simulink model "ejh68a"  (Simulink 3.00)
settings: Solver=ode5  StartTime=0.0  StopTime=30.0  FixedStep=0.1  MaxStep=0.001  RelTol=1e-3
undefined symbols (not defined in the file or in its folder): nonlinear
settings Model: LastModifiedBy=Administrador

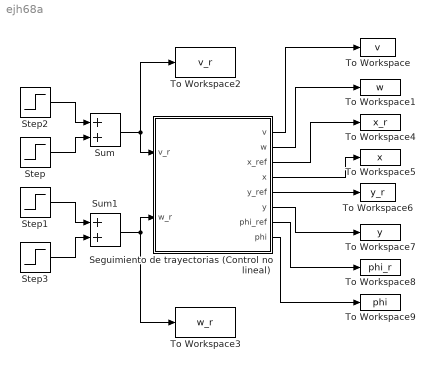
== system ejh68a ==
  Seguimiento de trayectorias (Control no lineal) : Subsystem  mask(Seguimiento de trayectorias empleando una ley de control no lineal){b=13.75, d=0.9, K2=19, x_inicial=1, y_inicial=0.5, phi_inicial=pi/6, x_r_inicial=0, y_r_inicial=0, phi_r_inicial=0}
      mask prompts: b "Parámetro beta:"; d "Parámetro delta:"; K2 "Parámetro K2:"; x_inicial "Coordenada x inicial del robot:"; y_inicial "Coordenada y inicial del robot:"; phi_inicial "Valor inicial de la orientación del robot (rad):"; x_r_inicial "Coordenada x inicial de la referencia:"; y_r_inicial "Coordenada y inicial de la referencia:"; phi_r_inicial "Orientación inicial de la referencia (rad):"
      mask help:
      | Este bloque permite simular una estrategia de control no lineal para el seguimiento de trayectorias. A la entrada se dispone de las velocidades lineal y angular de referencia. Se supone un cierto modelo para el vehículo.
      | El usuario puede modificar este bloque para introducir como referencia las coordenadas (x,y) y la orientación deseadas.
  Step : Step  Time=0  Before=0  After=0.2  SampleTime=0
  Step1 : Step  Time=0  Before=0  After=0.3  SampleTime=0
  Step2 : Step  Time=20  Before=0  After=-0.1  SampleTime=0
  Step3 : Step  Time=10  Before=0  After=-0.1  SampleTime=0
  Sum : Sum  Inputs=++  SaturateOnIntegerOverflow=on
  Sum1 : Sum  Inputs=++  SaturateOnIntegerOverflow=on
  To Workspace : ToWorkspace  VariableName=v  SampleTime=-1  SaveFormat=Matrix
  To Workspace1 : ToWorkspace  VariableName=w  SampleTime=-1  SaveFormat=Matrix
  To Workspace2 : ToWorkspace  VariableName=v_r  SampleTime=-1  SaveFormat=Matrix
  To Workspace3 : ToWorkspace  VariableName=w_r  SampleTime=-1  SaveFormat=Matrix
  To Workspace4 : ToWorkspace  VariableName=x_r  SampleTime=-1  SaveFormat=Matrix
  To Workspace5 : ToWorkspace  VariableName=x  SampleTime=-1  SaveFormat=Matrix
  To Workspace6 : ToWorkspace  VariableName=y_r  SampleTime=-1  SaveFormat=Matrix
  To Workspace7 : ToWorkspace  VariableName=y  SampleTime=-1  SaveFormat=Matrix
  To Workspace8 : ToWorkspace  VariableName=phi_r  SampleTime=-1  SaveFormat=Matrix
  To Workspace9 : ToWorkspace  VariableName=phi  SampleTime=-1  SaveFormat=Matrix
  wires:
  Step2/1 -> Sum/1
  Step/1 -> Sum/2
  Step1/1 -> Sum1/1
  Step3/1 -> Sum1/2
  Sum1/1 -> To Workspace3/1, Seguimiento de trayectorias (Control no lineal)/2(w_r)
  Sum/1 -> To Workspace2/1, Seguimiento de trayectorias (Control no lineal)/1(v_r)
  Seguimiento de trayectorias (Control no lineal)/1(v) -> To Workspace/1
  Seguimiento de trayectorias (Control no lineal)/2(w) -> To Workspace1/1
  Seguimiento de trayectorias (Control no lineal)/3(x_ref) -> To Workspace4/1
  Seguimiento de trayectorias (Control no lineal)/5(y_ref) -> To Workspace6/1
  Seguimiento de trayectorias (Control no lineal)/6(y) -> To Workspace7/1
  Seguimiento de trayectorias (Control no lineal)/7(phi_ref) -> To Workspace8/1
  Seguimiento de trayectorias (Control no lineal)/4(x) -> To Workspace5/1
  Seguimiento de trayectorias (Control no lineal)/8(phi) -> To Workspace9/1

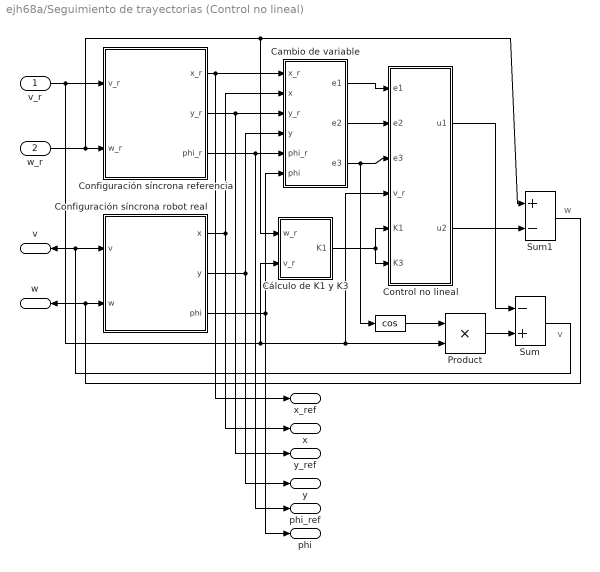
== system ejh68a/Seguimiento de trayectorias (Control no lineal) ==
  note: v
  note: w
  v_r : Inport  Port=1  PortWidth=-1  SampleTime=-1  DataType=auto
      settings: SignalType=auto
  w_r : Inport  Port=2  PortWidth=-1  SampleTime=-1  DataType=auto
      settings: SignalType=auto
  " " : Trigonometry  Operator=cos  OutputSignalType=auto
  Cambio de variable : Subsystem
  Configuración síncrona referencia : Subsystem
  Configuración síncrona robot real : Subsystem
  Control no lineal : Subsystem
  Cálculo de K1 y K3 : Subsystem
  Product : Product  Inputs=2  SaturateOnIntegerOverflow=on
  Sum : Sum  Inputs=-+  SaturateOnIntegerOverflow=on
  Sum1 : Sum  Inputs=+-  SaturateOnIntegerOverflow=on
  v : Outport  Orientation=left  Port=1
  w : Outport  Orientation=left  Port=2
  x_ref : Outport  Port=3
  x : Outport  Port=4
  y_ref : Outport  Port=5
  y : Outport  Port=6
  phi_ref : Outport  Port=7
  phi : Outport  Port=8
  wires:
  v_r/1 -> Configuración síncrona referencia/1(v_r), Product/2, Control no lineal/4(v_r), Cálculo de K1 y K3/2(v_r)
  " "/1 -> Product/1
  Product/1 -> Sum/2
  w_r/1 -> Configuración síncrona referencia/2(w_r), Sum1/1, Cálculo de K1 y K3/1(w_r)
  Sum1/1 -> Configuración síncrona robot real/2(w), w/1
  Sum/1 -> Configuración síncrona robot real/1(v), v/1
  Control no lineal/2(u2) -> Sum1/2
  Control no lineal/1(u1) -> Sum/1
  Cambio de variable/1(e1) -> Control no lineal/1(e1)
  Cambio de variable/2(e2) -> Control no lineal/2(e2)
  Cambio de variable/3(e3) -> " "/1, Control no lineal/3(e3)
  Cálculo de K1 y K3/1(K1) -> Control no lineal/5(K1), Control no lineal/6(K3)
  Configuración síncrona robot real/3(phi) -> Cambio de variable/6(phi), phi/1
  Configuración síncrona referencia/1(x_r) -> Cambio de variable/1(x_r), x_ref/1
  Configuración síncrona robot real/1(x) -> Cambio de variable/2(x), x/1
  Configuración síncrona referencia/2(y_r) -> Cambio de variable/3(y_r), y_ref/1
  Configuración síncrona robot real/2(y) -> Cambio de variable/4(y), y/1
  Configuración síncrona referencia/3(phi_r) -> Cambio de variable/5(phi_r), phi_ref/1

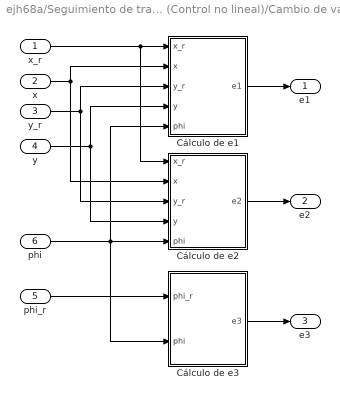
== system ejh68a/Seguimiento de trayectorias (Control no lineal)/Cambio de variable ==
  x_r : Inport  Port=1  PortWidth=-1  SampleTime=-1  DataType=auto
      settings: SignalType=auto
  x : Inport  Port=2  PortWidth=-1  SampleTime=-1  DataType=auto
      settings: SignalType=auto
  y_r : Inport  Port=3  PortWidth=-1  SampleTime=-1  DataType=auto
      settings: SignalType=auto
  y : Inport  Port=4  PortWidth=-1  SampleTime=-1  DataType=auto
      settings: SignalType=auto
  phi_r : Inport  Port=5  PortWidth=-1  SampleTime=-1  DataType=auto
      settings: SignalType=auto
  phi : Inport  Port=6  PortWidth=-1  SampleTime=-1  DataType=auto
      settings: SignalType=auto
  Cálculo de e1 : Subsystem
  Cálculo de e2 : Subsystem
  Cálculo de e3 : Subsystem
  e1 : Outport  Port=1
  e2 : Outport  Port=2
  e3 : Outport  Port=3
  wires:
  x_r/1 -> Cálculo de e1/1(x_r), Cálculo de e2/1(x_r)
  x/1 -> Cálculo de e1/2(x), Cálculo de e2/2(x)
  y_r/1 -> Cálculo de e1/3(y_r), Cálculo de e2/3(y_r)
  y/1 -> Cálculo de e1/4(y), Cálculo de e2/4(y)
  phi_r/1 -> Cálculo de e3/1(phi_r)
  phi/1 -> Cálculo de e2/5(phi), Cálculo de e3/2(phi), Cálculo de e1/5(phi)
  Cálculo de e1/1(e1) -> e1/1
  Cálculo de e2/1(e2) -> e2/1
  Cálculo de e3/1(e3) -> e3/1

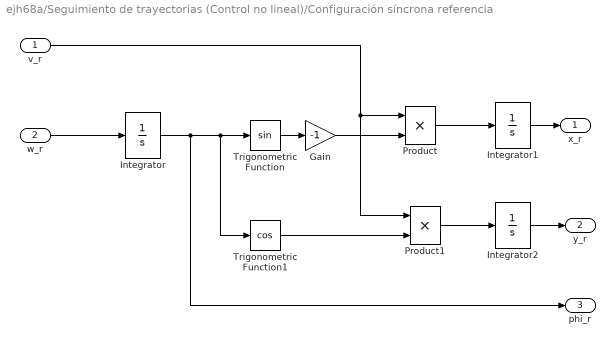
== system ejh68a/Seguimiento de trayectorias (Control no lineal)/Configuración síncrona referencia ==
  v_r : Inport  Port=1  PortWidth=-1  SampleTime=-1  DataType=auto
      settings: SignalType=auto
  w_r : Inport  Port=2  PortWidth=-1  SampleTime=-1  DataType=auto
      settings: SignalType=auto
  Gain : Gain  Gain=-1  SaturateOnIntegerOverflow=on
  Integrator : Integrator  ExternalReset=none  InitialConditionSource=internal  InitialCondition=phi_r_inicial  LimitOutput=off  UpperSaturationLimit=inf  LowerSaturationLimit=-inf  ShowSaturationPort=off  ShowStatePort=off  AbsoluteTolerance=auto
  Integrator1 : Integrator  ExternalReset=none  InitialConditionSource=internal  InitialCondition=x_r_inicial  LimitOutput=off  UpperSaturationLimit=inf  LowerSaturationLimit=-inf  ShowSaturationPort=off  ShowStatePort=off  AbsoluteTolerance=auto
  Integrator2 : Integrator  ExternalReset=none  InitialConditionSource=internal  InitialCondition=y_r_inicial  LimitOutput=off  UpperSaturationLimit=inf  LowerSaturationLimit=-inf  ShowSaturationPort=off  ShowStatePort=off  AbsoluteTolerance=auto
  Product : Product  Inputs=2  SaturateOnIntegerOverflow=on
  Product1 : Product  Inputs=2  SaturateOnIntegerOverflow=on
  Trigonometric Function : Trigonometry  Operator=sin  OutputSignalType=auto
  Trigonometric Function1 : Trigonometry  Operator=cos  OutputSignalType=auto
  x_r : Outport  Port=1
  y_r : Outport  Port=2
  phi_r : Outport  Port=3
  wires:
  Product1/1 -> Integrator2/1
  Product/1 -> Integrator1/1
  Integrator/1 -> Trigonometric Function/1, Trigonometric Function1/1, phi_r/1
  Integrator1/1 -> x_r/1
  Integrator2/1 -> y_r/1
  v_r/1 -> Product/1, Product1/1
  w_r/1 -> Integrator/1
  Gain/1 -> Product/2
  Trigonometric Function/1 -> Gain/1
  Trigonometric Function1/1 -> Product1/2

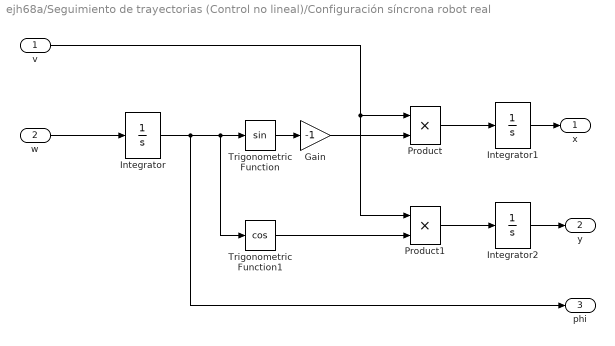
== system ejh68a/Seguimiento de trayectorias (Control no lineal)/Configuración síncrona robot real ==
  v : Inport  Port=1  PortWidth=-1  SampleTime=-1  DataType=auto
      settings: SignalType=auto
  w : Inport  Port=2  PortWidth=-1  SampleTime=-1  DataType=auto
      settings: SignalType=auto
  Gain : Gain  Gain=-1  SaturateOnIntegerOverflow=on
  Integrator : Integrator  ExternalReset=none  InitialConditionSource=internal  InitialCondition=phi_inicial  LimitOutput=off  UpperSaturationLimit=inf  LowerSaturationLimit=-inf  ShowSaturationPort=off  ShowStatePort=off  AbsoluteTolerance=auto
  Integrator1 : Integrator  ExternalReset=none  InitialConditionSource=internal  InitialCondition=x_inicial  LimitOutput=off  UpperSaturationLimit=inf  LowerSaturationLimit=-inf  ShowSaturationPort=off  ShowStatePort=off  AbsoluteTolerance=auto
  Integrator2 : Integrator  ExternalReset=none  InitialConditionSource=internal  InitialCondition=y_inicial  LimitOutput=off  UpperSaturationLimit=inf  LowerSaturationLimit=-inf  ShowSaturationPort=off  ShowStatePort=off  AbsoluteTolerance=auto
  Product : Product  Inputs=2  SaturateOnIntegerOverflow=on
  Product1 : Product  Inputs=2  SaturateOnIntegerOverflow=on
  Trigonometric Function : Trigonometry  Operator=sin  OutputSignalType=auto
  Trigonometric Function1 : Trigonometry  Operator=cos  OutputSignalType=auto
  x : Outport  Port=1
  y : Outport  Port=2
  phi : Outport  Port=3
  wires:
  Product1/1 -> Integrator2/1
  Product/1 -> Integrator1/1
  Gain/1 -> Product/2
  Integrator/1 -> Trigonometric Function/1, Trigonometric Function1/1, phi/1
  Integrator1/1 -> x/1
  Integrator2/1 -> y/1
  v/1 -> Product/1, Product1/1
  w/1 -> Integrator/1
  Trigonometric Function/1 -> Gain/1
  Trigonometric Function1/1 -> Product1/2

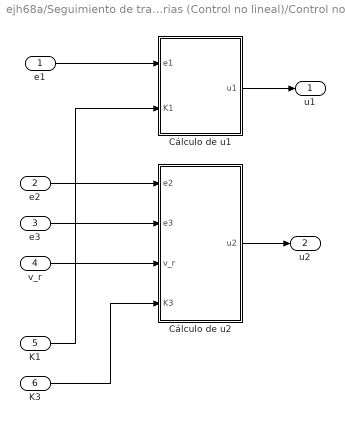
== system ejh68a/Seguimiento de trayectorias (Control no lineal)/Control no lineal ==
  e1 : Inport  Port=1  PortWidth=-1  SampleTime=-1  DataType=auto
      settings: SignalType=auto
  e2 : Inport  Port=2  PortWidth=-1  SampleTime=-1  DataType=auto
      settings: SignalType=auto
  e3 : Inport  Port=3  PortWidth=-1  SampleTime=-1  DataType=auto
      settings: SignalType=auto
  v_r : Inport  Port=4  PortWidth=-1  SampleTime=-1  DataType=auto
      settings: SignalType=auto
  K1 : Inport  Port=5  PortWidth=-1  SampleTime=-1  DataType=auto
      settings: SignalType=auto
  K3 : Inport  Port=6  PortWidth=-1  SampleTime=-1  DataType=auto
      settings: SignalType=auto
  Cálculo de u1 : Subsystem
  "Cálculo de u2 " : Subsystem
  u1 : Outport  Port=1
  u2 : Outport  Port=2
  wires:
  e1/1 -> Cálculo de u1/1(e1)
  e2/1 -> "Cálculo de u2 "/1(e2)
  e3/1 -> "Cálculo de u2 "/2(e3)
  Cálculo de u1/1(u1) -> u1/1
  "Cálculo de u2 "/1(u2) -> u2/1
  v_r/1 -> "Cálculo de u2 "/3(v_r)
  K1/1 -> Cálculo de u1/2(K1)
  K3/1 -> "Cálculo de u2 "/4(K3)

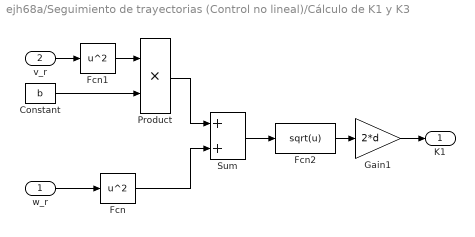
== system ejh68a/Seguimiento de trayectorias (Control no lineal)/Cálculo de K1 y K3 ==
  w_r : Inport  Port=1  PortWidth=-1  SampleTime=-1  DataType=auto
      settings: SignalType=auto
  v_r : Inport  Port=2  PortWidth=-1  SampleTime=-1  DataType=auto
      settings: SignalType=auto
  Constant : Constant  Value=b
  Fcn : Fcn  Expr=u^2
  Fcn1 : Fcn  Expr=u^2
  Fcn2 : Fcn  Expr=sqrt(u)
  Gain1 : Gain  Gain=2*d  SaturateOnIntegerOverflow=on
  Product : Product  Inputs=2  SaturateOnIntegerOverflow=on
  Sum : Sum  Inputs=++  SaturateOnIntegerOverflow=on
  K1 : Outport  Port=1
  wires:
  w_r/1 -> Fcn/1
  v_r/1 -> Fcn1/1
  Fcn1/1 -> Product/1
  Constant/1 -> Product/2
  Product/1 -> Sum/1
  Fcn/1 -> Sum/2
  Sum/1 -> Fcn2/1
  Fcn2/1 -> Gain1/1
  Gain1/1 -> K1/1

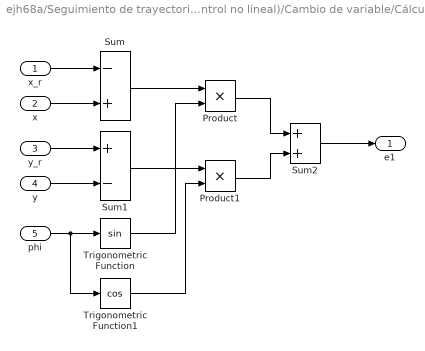
== system ejh68a/Seguimiento de trayectorias (Control no lineal)/Cambio de variable/Cálculo de e1 ==
  x_r : Inport  Port=1  PortWidth=-1  SampleTime=-1  DataType=auto
      settings: SignalType=auto
  x : Inport  Port=2  PortWidth=-1  SampleTime=-1  DataType=auto
      settings: SignalType=auto
  y_r : Inport  Port=3  PortWidth=-1  SampleTime=-1  DataType=auto
      settings: SignalType=auto
  y : Inport  Port=4  PortWidth=-1  SampleTime=-1  DataType=auto
      settings: SignalType=auto
  phi : Inport  Port=5  PortWidth=-1  SampleTime=-1  DataType=auto
      settings: SignalType=auto
  Product : Product  Inputs=2  SaturateOnIntegerOverflow=on
  Product1 : Product  Inputs=2  SaturateOnIntegerOverflow=on
  Sum : Sum  Inputs=-+  SaturateOnIntegerOverflow=on
  Sum1 : Sum  Inputs=+-  SaturateOnIntegerOverflow=on
  Sum2 : Sum  Inputs=++  SaturateOnIntegerOverflow=on
  Trigonometric Function : Trigonometry  Operator=sin  OutputSignalType=auto
  Trigonometric Function1 : Trigonometry  Operator=cos  OutputSignalType=auto
  e1 : Outport  Port=1
  wires:
  x_r/1 -> Sum/1
  x/1 -> Sum/2
  y_r/1 -> Sum1/1
  y/1 -> Sum1/2
  phi/1 -> Trigonometric Function/1, Trigonometric Function1/1
  Sum/1 -> Product/1
  Trigonometric Function/1 -> Product/2
  Sum1/1 -> Product1/1
  Trigonometric Function1/1 -> Product1/2
  Product/1 -> Sum2/1
  Product1/1 -> Sum2/2
  Sum2/1 -> e1/1

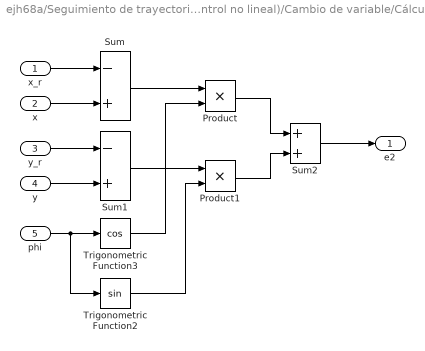
== system ejh68a/Seguimiento de trayectorias (Control no lineal)/Cambio de variable/Cálculo de e2 ==
  x_r : Inport  Port=1  PortWidth=-1  SampleTime=-1  DataType=auto
      settings: SignalType=auto
  x : Inport  Port=2  PortWidth=-1  SampleTime=-1  DataType=auto
      settings: SignalType=auto
  y_r : Inport  Port=3  PortWidth=-1  SampleTime=-1  DataType=auto
      settings: SignalType=auto
  y : Inport  Port=4  PortWidth=-1  SampleTime=-1  DataType=auto
      settings: SignalType=auto
  phi : Inport  Port=5  PortWidth=-1  SampleTime=-1  DataType=auto
      settings: SignalType=auto
  Product : Product  Inputs=2  SaturateOnIntegerOverflow=on
  Product1 : Product  Inputs=2  SaturateOnIntegerOverflow=on
  Sum : Sum  Inputs=-+  SaturateOnIntegerOverflow=on
  Sum1 : Sum  Inputs=-+  SaturateOnIntegerOverflow=on
  Sum2 : Sum  Inputs=++  SaturateOnIntegerOverflow=on
  Trigonometric Function2 : Trigonometry  Operator=sin  OutputSignalType=auto
  Trigonometric Function3 : Trigonometry  Operator=cos  OutputSignalType=auto
  e2 : Outport  Port=1
  wires:
  x_r/1 -> Sum/1
  x/1 -> Sum/2
  y_r/1 -> Sum1/1
  y/1 -> Sum1/2
  phi/1 -> Trigonometric Function3/1, Trigonometric Function2/1
  Sum/1 -> Product/1
  Trigonometric Function3/1 -> Product/2
  Sum1/1 -> Product1/1
  Trigonometric Function2/1 -> Product1/2
  Product/1 -> Sum2/1
  Product1/1 -> Sum2/2
  Sum2/1 -> e2/1

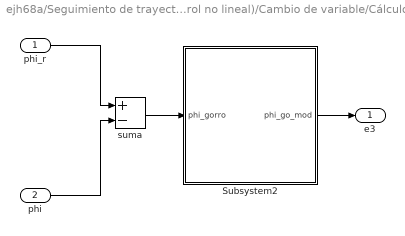
== system ejh68a/Seguimiento de trayectorias (Control no lineal)/Cambio de variable/Cálculo de e3 ==
  phi_r : Inport  Port=1  PortWidth=-1  SampleTime=-1  DataType=auto
      settings: SignalType=auto
  phi : Inport  Port=2  PortWidth=-1  SampleTime=-1  DataType=auto
      settings: SignalType=auto
  Subsystem2 : Subsystem
      mask Description: Pasa phi gorro al intervalo -180,180
  suma : Sum  Inputs=+-  SaturateOnIntegerOverflow=on
  e3 : Outport  Port=1
  wires:
  phi/1 -> suma/2
  phi_r/1 -> suma/1
  suma/1 -> Subsystem2/1(phi_gorro)
  Subsystem2/1(phi_go_mod) -> e3/1

== system ejh68a/Seguimiento de trayectorias (Control no lineal)/Control no lineal/Cálculo de u1 ==
  e1 : Inport  Port=1  PortWidth=-1  SampleTime=-1  DataType=auto
      settings: SignalType=auto
  K1 : Inport  Port=2  PortWidth=-1  SampleTime=-1  DataType=auto
      settings: SignalType=auto
  Gain : Gain  Gain=-1  SaturateOnIntegerOverflow=on
  Product : Product  Inputs=2  SaturateOnIntegerOverflow=on
  u1 : Outport  Port=1
  wires:
  e1/1 -> Product/1
  Product/1 -> u1/1
  K1/1 -> Gain/1
  Gain/1 -> Product/2

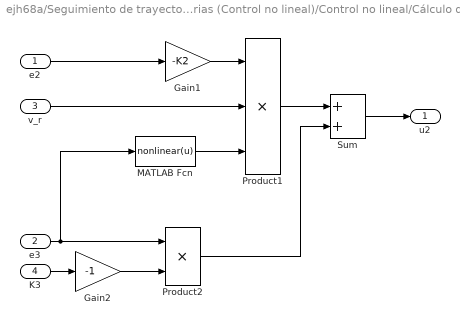
== system ejh68a/Seguimiento de trayectorias (Control no lineal)/Control no lineal/Cálculo de u2  ==
  e2 : Inport  Port=1  PortWidth=-1  SampleTime=-1  DataType=auto
      settings: SignalType=auto
  e3 : Inport  Port=2  PortWidth=-1  SampleTime=-1  DataType=auto
      settings: SignalType=auto
  v_r : Inport  Port=3  PortWidth=-1  SampleTime=-1  DataType=auto
      settings: SignalType=auto
  K3 : Inport  Port=4  PortWidth=-1  SampleTime=-1  DataType=auto
      settings: SignalType=auto
  Gain1 : Gain  Gain=-K2  SaturateOnIntegerOverflow=on
  Gain2 : Gain  Gain=-1  SaturateOnIntegerOverflow=on
  MATLAB Fcn : MATLABFcn  MATLABFcn=nonlinear(u)  OutputWidth=-1  OutputSignalType=auto
  Product1 : Product  Inputs=3  SaturateOnIntegerOverflow=on
  Product2 : Product  Inputs=2  SaturateOnIntegerOverflow=on
  Sum : Sum  Inputs=++  SaturateOnIntegerOverflow=on
  u2 : Outport  Port=1
  wires:
  MATLAB Fcn/1 -> Product1/3
  Gain1/1 -> Product1/1
  Product1/1 -> Sum/1
  Sum/1 -> u2/1
  e2/1 -> Gain1/1
  K3/1 -> Gain2/1
  Gain2/1 -> Product2/2
  Product2/1 -> Sum/2
  v_r/1 -> Product1/2
  e3/1 -> MATLAB Fcn/1, Product2/1

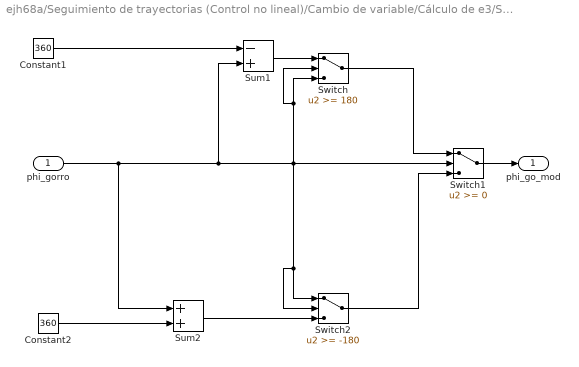
== system ejh68a/Seguimiento de trayectorias (Control no lineal)/Cambio de variable/Cálculo de e3/Subsystem2 ==
  phi_gorro : Inport  Port=1  PortWidth=-1  SampleTime=-1  DataType=auto
      settings: SignalType=auto
  Constant1 : Constant  Value=360
  Constant2 : Constant  Value=360
  Sum1 : Sum  Inputs=-+  SaturateOnIntegerOverflow=on
  Sum2 : Sum  Inputs=++  SaturateOnIntegerOverflow=on
  Switch : Switch  Threshold=180
  Switch1 : Switch  Threshold=0
  Switch2 : Switch  Threshold=-180
  phi_go_mod : Outport  Port=1
  wires:
  Switch1/1 -> phi_go_mod/1
  Switch/1 -> Switch1/1
  Switch2/1 -> Switch1/3
  Constant1/1 -> Sum1/1
  Sum1/1 -> Switch/1
  Sum2/1 -> Switch2/3
  phi_gorro/1 -> Sum1/2, Switch1/2, Switch/3, Switch/2, Switch2/1, Switch2/2, Sum2/1
  Constant2/1 -> Sum2/2
